simulink model "oldCubesatFullSim"  (R2024a)
settings: Solver=FixedStepAuto  StartTime=0.0  StopTime=7200  FixedStep=0.01  MaxStep=1  MinStep=0.001  RelTol=1e-3
libraries: sharedtransform x2, simulink_extras x2, aerolibutil x1
settings Model: Creator=samuel  LastModifiedBy=joshu
settings OptimizationCC: ReuseModelBlockBuffer=off
settings ModelReferenceCC: EnableRefExpFcnMdlSchedulingChecks=on
settings RTWCC: GPUComputeCapability=3.5

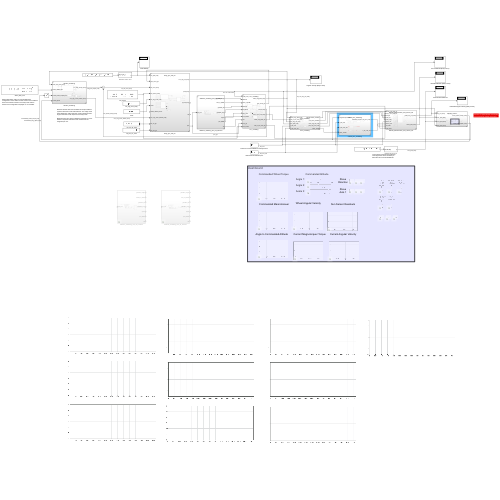
[thumbnail: Simulink's stored preview of the top-level diagram]
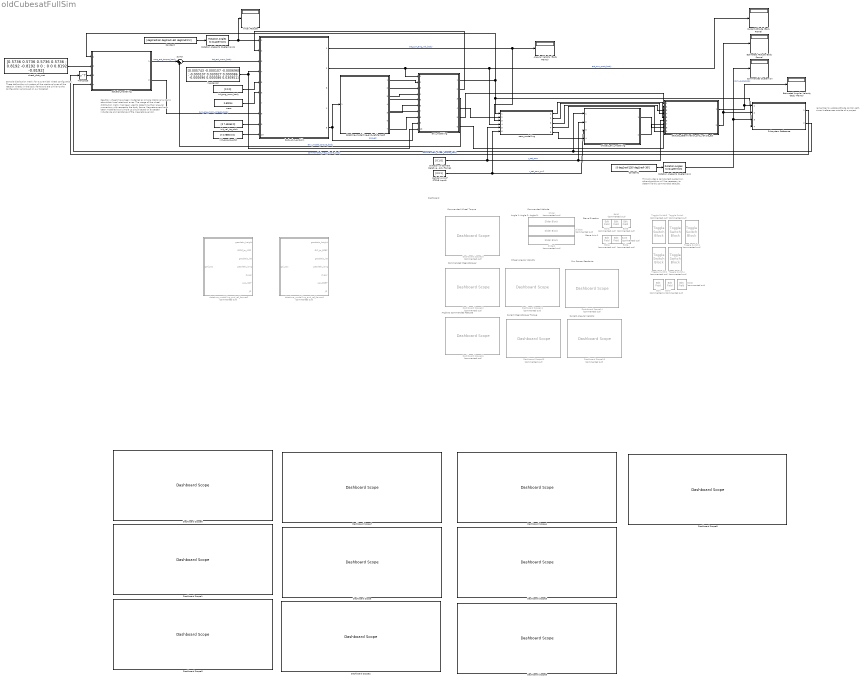
== system oldCubesatFullSim ==
  note: remember to update attitude control path,
      | since it references outside of a project
  note: This provides a sample test quaternion, other algorithms will be necessary to determine this commanded attitude.
  note: Reaction wheels have been modelled as simple rotational systems about their local rotational axes. The usage of the wheel distribution matrix has been used to determine their angular momentum with respect to the body frame.
      |
      | Magnetorquers have been modelled as a simple LC circuit based on expected inductance and resistance of the magnetorquer coil.
  note: Sample distribution matrix for a pyramidal wheel configuration. These define the unit vectors of the rotational axes of the reaction wheels in the body frame and are similar to the configuration employed on our CubeSat.
  note: Commanded Wheel Torque
  note: Angle to Commanded Attitude
  note: Dashboard
  note: Wheel Angular Velocity
  note: Commanded Attitude
  note: Commanded Magnotorquer
  note: Steve Axis 1
  note: Angle 1:
      |
      | Angle 2:
      |
      | Angle 3:
  note: Current Angular Velocity
  note: Steve Direction
  note: Current Magnotorquer Torque
  note: Sun Sensor Readouts
  Angular Velocity (Body Frame) : Display
  Commanded Quaternion : Display
  Constant : Constant  Value=[deg2rad(34) deg2rad(-63) deg2rad(21)]
  Constant1 : Constant  Value=[0 deg2rad(135) deg2rad(-30)]
  Current Attitude (Body Frame) : Display
  Dashboard Scope{,1..9} (10 alike) : DashboardScope
  Dashboard Scope10 : DashboardScope  Commented=on  Ymin=0  NormalizeYAxis=on  TicksPosition=Inside
  Dashboard Scope{11..15} (5 alike) : DashboardScope  Commented=on  TicksPosition=Inside
  Dashboard Scope16 : DashboardScope  Commented=on  Ymin=0  UpdateMode=Scroll  NormalizeYAxis=on  TicksPosition=Inside
  Direction of Camera Relative to Body Frame1 : Constant  Value=[0 1 0]
  Edit{,1..8} (9 alike) : EditField  Commented=on  LabelPosition=Hide  ShowInitialText=on  Alignment=Center
  Estimated Angular Velocity (Body Frame) : Display
  Estimated Attitude (Body Frame) : Display
  Initial Attitude : Display
  Rotation Angles to Quaternions : sharedtransform/Rotation Angles to Quaternions  rotationOrder=ZYX  aMode=aMode
  Rotation Angles to Quaternions1 : sharedtransform/Rotation Angles to Quaternions  rotationOrder=ZYX  aMode=aMode
  Slider : SliderBlock  Commented=on  LabelPosition=Hide  ScaleMin=-3.1415  ScaleMax=3.1415
  Slider1 : SliderBlock  Commented=on  LabelPosition=Hide  ScaleMin=-3.1415  ScaleMax=3.1415
  Slider2 : SliderBlock  Commented=on  LabelPosition=Hide  ScaleMin=-3.1415  ScaleMax=3.1415
  Subsystem Reference : Subsystem  ReferencedSubsystem=attitude_control
  Sum3 : Sum  Inputs=|++
  Toggle Switch{,1..4} (5 alike) : ToggleSwitchBlock  Commented=on
      settings: Values={{'Off', 'On'}, [0 1]}
  Transpose : Math  Operator=transpose
  Vertical Axis of STEVE Input1 : Constant  Value=[0 0 1]
  actuator_modelling : Subsystem  ReferencedSubsystem=actuator_modelling
  attitude_determination_and_vehicle_est : Subsystem  ReferencedSubsystem=attitude_determination_and_vehicle_est
  body_dyn_and_kin : Subsystem  ReferencedSubsystem=body_dyn_and_kin
  datetime_modelling_and_ref_frames1 : Subsystem  Commented=on
  datetime_modelling_and_ref_frames2 : Subsystem  Commented=on
  datetime_modelling_and_ref_frames3 : Subsystem  ReferencedSubsystem=datetime_modelling_and_ref_frames
  env_modelling : Subsystem  ReferencedSubsystem=env_modelling
  iner_tensor : Constant  Value=[0.005743 -0.000107 -0.0006965 ; -0.000107 0.030927 0.000086 ; -0.000696 0.000086 0.030951]
  init_ang_mom_body : Constant  Value=[0 0 0]
  init_pos_iss_orbit : Constant  Value=[7.178e6 0 0]
  init_vel_iss_orbit : Constant  Value=[0 7.452e3 0]
  mass : Constant  Value=2.60014
  onboad_env_modelling : Subsystem  ReferencedSubsystem=onboad_env_modelling
  sens_modelling : Subsystem  ReferencedSubsystem=sens_modelling
  wheel_distr_mat : Constant  Value=[0.5736 0.5736 0.5736 0.5736 ; 0.8192 -0.8192 0 0 ; 0 0 0.8192 -0.8192]
  wires:
  iner_tensor/1 -> env_modelling/10, body_dyn_and_kin/4
  wheel_distr_mat/1 -> actuator_modelling/2
  actuator_modelling/1 -> Sum3/1  "mag_act_torque_body"
  body_dyn_and_kin/2 -> sens_modelling/4, Current Attitude (Body Frame)/1, env_modelling/1  "act_curr_quat_body"
  body_dyn_and_kin/5 -> datetime_modelling_and_ref_frames3/1, env_modelling/9  "pos_gci"
  Sum3/1 -> body_dyn_and_kin/3  "tot_ext_mom_body"
  init_ang_mom_body/1 -> body_dyn_and_kin/5
  mass/1 -> body_dyn_and_kin/6
  actuator_modelling/2 -> body_dyn_and_kin/8  "curr_ang_mom_wheels_body"
  init_vel_iss_orbit/1 -> body_dyn_and_kin/9
  init_pos_iss_orbit/1 -> body_dyn_and_kin/10
  env_modelling/1 -> sens_modelling/1, Subsystem Reference/4, actuator_modelling/1
  datetime_modelling_and_ref_frames3/1 -> env_modelling/2
  datetime_modelling_and_ref_frames3/2 -> env_modelling/3
  datetime_modelling_and_ref_frames3/3 -> env_modelling/4
  datetime_modelling_and_ref_frames3/4 -> env_modelling/5
  datetime_modelling_and_ref_frames3/5 -> env_modelling/6
  datetime_modelling_and_ref_frames3/6 -> env_modelling/7
  datetime_modelling_and_ref_frames3/7 -> env_modelling/8
  env_modelling/2 -> body_dyn_and_kin/2
  env_modelling/3 -> Sum3/2  "env_model_torque_body"
  env_modelling/4 -> sens_modelling/2
  attitude_determination_and_vehicle_est/1 -> Estimated Angular Velocity (Body Frame)/1, Subsystem Reference/1
  attitude_determination_and_vehicle_est/2 -> Estimated Attitude (Body Frame)/1, Subsystem Reference/2
  Subsystem Reference/1 -> Transpose/1  "commanded_wheel_torque_body"
  body_dyn_and_kin/1 -> sens_modelling/3, Angular Velocity (Body Frame)/1  "act_curr_ang_vel_body"
  sens_modelling/1 -> attitude_determination_and_vehicle_est/5
  sens_modelling/2 -> attitude_determination_and_vehicle_est/4
  env_modelling/5 -> attitude_determination_and_vehicle_est/1
  env_modelling/6 -> attitude_determination_and_vehicle_est/2
  Transpose/1 -> actuator_modelling/3
  Constant1/1 -> Rotation Angles to Quaternions/1
  Rotation Angles to Quaternions/1 -> Subsystem Reference/3, Commanded Quaternion/1  "com_quat_body"
  Rotation Angles to Quaternions1/1 -> body_dyn_and_kin/1, Initial Attitude/1
  Constant/1 -> Rotation Angles to Quaternions1/1
  Subsystem Reference/2 -> actuator_modelling/4, onboad_env_modelling/1  "commanded_mag_dipole_body"
  Direction of Camera Relative to Body Frame1/1 -> onboad_env_modelling/2, attitude_determination_and_vehicle_est/6, sens_modelling/5  "r_sat_com"
  Vertical Axis of STEVE Input1/1 -> sens_modelling/6, onboad_env_modelling/3  "r_sat_com_ax1"
  sens_modelling/3 -> attitude_determination_and_vehicle_est/3
  sens_modelling/5 -> onboad_env_modelling/4
  onboad_env_modelling/2 -> attitude_determination_and_vehicle_est/7
  onboad_env_modelling/1 -> attitude_determination_and_vehicle_est/8
  sens_modelling/4 -> attitude_determination_and_vehicle_est/9

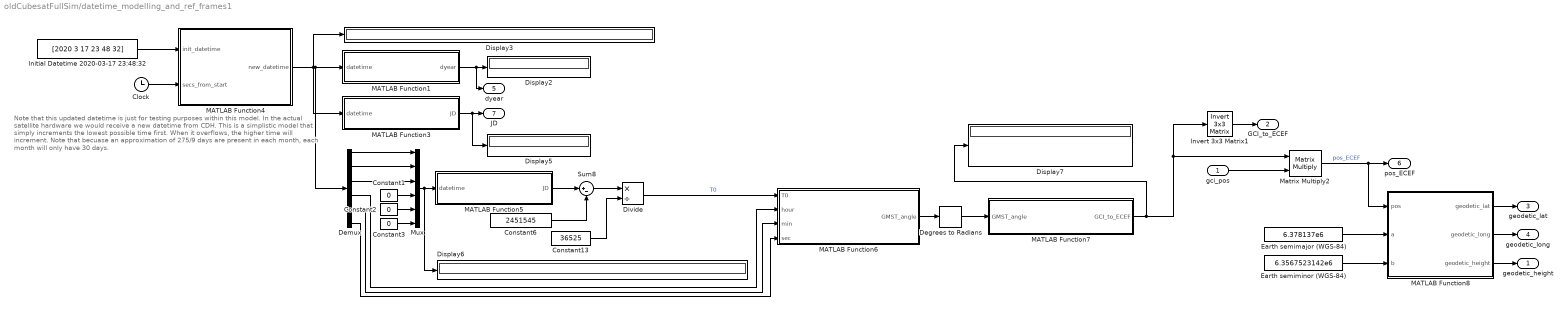
== system oldCubesatFullSim/datetime_modelling_and_ref_frames1 ==
  note: Note that this updated datetime is just for testing purposes within this model. In the actual satellite hardware we would receive a new datetime from CDH. This is a simplistic model that simply increments the lowest possible time first. When it overflows, the higher time will increment. Note that becuase an approximation of 275/9 days are present in each month, each month will only have 30 days.
  gci_pos : Inport
  Clock : Clock
  Constant1 : Constant  Value=0
  Constant13 : Constant  Value=36525
  Constant2 : Constant  Value=0
  Constant3 : Constant  Value=0
  Constant6 : Constant  Value=2451545
  Degrees to Radians : simulink_extras/Transformations/Degrees to Radians
  Demux : Demux  Outputs=6
  Display{2..3,5..7} (5 alike) : Display
  Divide : Product  Inputs=*/
  Earth semimajor (WGS-84) : Constant  Value=6.378137e6
  Earth semiminor (WGS-84) : Constant  Value=6.3567523142e6
  Initial Datetime 2020-03-17 23:48:32 : Constant  Value=[2020 3 17 23 48 32]
  Invert 3x3 Matrix1 : aerolibutil/Invert  3x3 Matrix
  MATLAB Function1 : MATLAB Function  TreatAsAtomicUnit=on
  MATLAB Function3 : MATLAB Function  TreatAsAtomicUnit=on
  MATLAB Function4 : MATLAB Function  TreatAsAtomicUnit=on
  MATLAB Function5 : MATLAB Function  TreatAsAtomicUnit=on
  MATLAB Function6 : MATLAB Function  TreatAsAtomicUnit=on
  MATLAB Function7 : MATLAB Function  TreatAsAtomicUnit=on
  MATLAB Function8 : MATLAB Function  TreatAsAtomicUnit=on
  Matrix Multiply2 : Product  Multiplication=Matrix(*)
  Mux : Mux  Inputs=6
  Sum8 : Sum  Inputs=|+-
  geodetic_height : Outport
  GCI_to_ECEF : Outport  Port=2
  geodetic_lat : Outport  Port=3
  geodetic_long : Outport  Port=4
  dyear : Outport  Port=5
  pos_ECEF : Outport  Port=6
  JD : Outport  Port=7
  wires:
  Constant3/1 -> Mux/6
  MATLAB Function8/1(geodetic_lat) -> geodetic_lat/1
  Divide/1 -> MATLAB Function6/1(T0)  "T0"
  MATLAB Function4/1(new_datetime) -> Demux/1, MATLAB Function1/1(datetime), MATLAB Function3/1(datetime), Display3/1
  MATLAB Function6/1(GMST_angle) -> Degrees to Radians/1
  MATLAB Function1/1(dyear) -> dyear/1, Display2/1
  Invert 3x3 Matrix1/1 -> GCI_to_ECEF/1
  MATLAB Function3/1(JD) -> Display5/1, JD/1
  MATLAB Function8/3(geodetic_height) -> geodetic_height/1
  MATLAB Function8/2(geodetic_long) -> geodetic_long/1
  Constant1/1 -> Mux/4
  Demux/5 -> MATLAB Function6/3(min)
  Demux/1 -> Mux/1
  Sum8/1 -> Divide/1
  Constant13/1 -> Divide/2
  Earth semiminor (WGS-84)/1 -> MATLAB Function8/3(b)
  Earth semimajor (WGS-84)/1 -> MATLAB Function8/2(a)
  Matrix Multiply2/1 -> MATLAB Function8/1(pos), pos_ECEF/1  "pos_ECEF"
  Demux/6 -> MATLAB Function6/4(sec)
  Constant6/1 -> Sum8/2
  gci_pos/1 -> Matrix Multiply2/2
  MATLAB Function5/1(JD) -> Sum8/1
  MATLAB Function7/1(GCI_to_ECEF) -> Matrix Multiply2/1, Invert 3x3 Matrix1/1, Display7/1
  Degrees to Radians/1 -> MATLAB Function7/1(GMST_angle)
  Mux/1 -> Display6/1, MATLAB Function5/1(datetime)
  Initial Datetime 2020-03-17 23:48:32/1 -> MATLAB Function4/1(init_datetime)
  Clock/1 -> MATLAB Function4/2(secs_from_start)
  Demux/3 -> Mux/3
  Demux/4 -> MATLAB Function6/2(hour)
  Demux/2 -> Mux/2
  Constant2/1 -> Mux/5

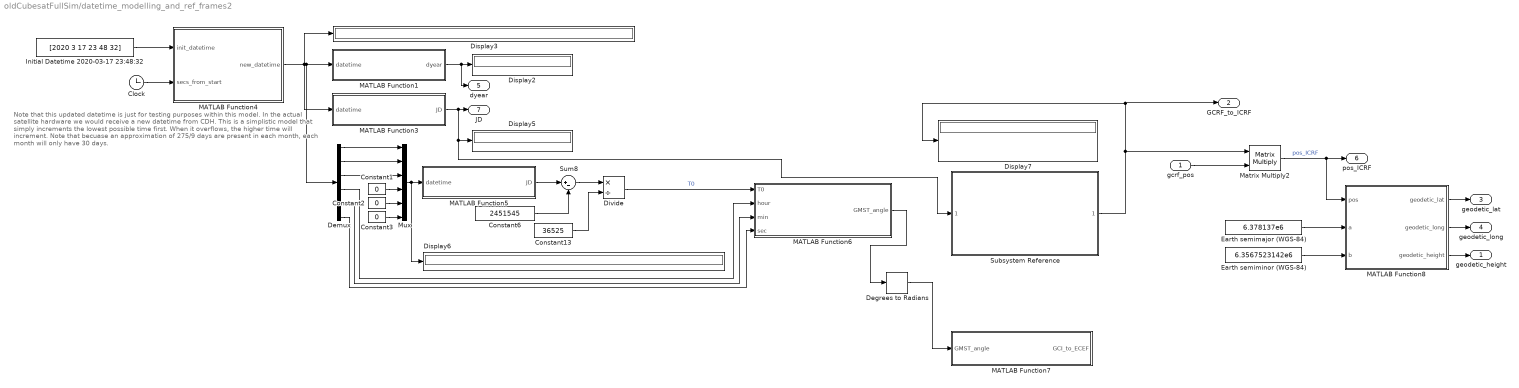
== system oldCubesatFullSim/datetime_modelling_and_ref_frames2 ==
  note: Note that this updated datetime is just for testing purposes within this model. In the actual satellite hardware we would receive a new datetime from CDH. This is a simplistic model that simply increments the lowest possible time first. When it overflows, the higher time will increment. Note that becuase an approximation of 275/9 days are present in each month, each month will only have 30 days.
  gcrf_pos : Inport
  Clock : Clock
  Constant1 : Constant  Value=0
  Constant13 : Constant  Value=36525
  Constant2 : Constant  Value=0
  Constant3 : Constant  Value=0
  Constant6 : Constant  Value=2451545
  Degrees to Radians : simulink_extras/Transformations/Degrees to Radians
  Demux : Demux  Outputs=6
  Display{2..3,5..7} (5 alike) : Display
  Divide : Product  Inputs=*/
  Earth semimajor (WGS-84) : Constant  Value=6.378137e6
  Earth semiminor (WGS-84) : Constant  Value=6.3567523142e6
  Initial Datetime 2020-03-17 23:48:32 : Constant  Value=[2020 3 17 23 48 32]
  MATLAB Function1 : MATLAB Function  TreatAsAtomicUnit=on
  MATLAB Function3 : MATLAB Function  TreatAsAtomicUnit=on
  MATLAB Function4 : MATLAB Function  TreatAsAtomicUnit=on
  MATLAB Function5 : MATLAB Function  TreatAsAtomicUnit=on
  MATLAB Function6 : MATLAB Function  TreatAsAtomicUnit=on
  MATLAB Function7 : MATLAB Function  TreatAsAtomicUnit=on
  MATLAB Function8 : MATLAB Function  TreatAsAtomicUnit=on
  Matrix Multiply2 : Product  Multiplication=Matrix(*)
  Mux : Mux  Inputs=6
  Subsystem Reference : Subsystem  ReferencedSubsystem=GCRF_to_ICRF
  Sum8 : Sum  Inputs=|+-
  geodetic_height : Outport
  GCRF_to_ICRF : Outport  Port=2
  geodetic_lat : Outport  Port=3
  geodetic_long : Outport  Port=4
  dyear : Outport  Port=5
  pos_ICRF : Outport  Port=6
  JD : Outport  Port=7
  wires:
  Constant3/1 -> Mux/6
  MATLAB Function8/1(geodetic_lat) -> geodetic_lat/1
  Divide/1 -> MATLAB Function6/1(T0)  "T0"
  MATLAB Function4/1(new_datetime) -> Demux/1, MATLAB Function1/1(datetime), MATLAB Function3/1(datetime), Display3/1
  MATLAB Function6/1(GMST_angle) -> Degrees to Radians/1
  MATLAB Function1/1(dyear) -> dyear/1, Display2/1
  MATLAB Function3/1(JD) -> Subsystem Reference/1, Display5/1, JD/1
  MATLAB Function8/3(geodetic_height) -> geodetic_height/1
  MATLAB Function8/2(geodetic_long) -> geodetic_long/1
  Constant1/1 -> Mux/4
  Demux/5 -> MATLAB Function6/3(min)
  Demux/1 -> Mux/1
  Sum8/1 -> Divide/1
  Constant13/1 -> Divide/2
  Earth semiminor (WGS-84)/1 -> MATLAB Function8/3(b)
  Earth semimajor (WGS-84)/1 -> MATLAB Function8/2(a)
  Matrix Multiply2/1 -> MATLAB Function8/1(pos), pos_ICRF/1  "pos_ICRF"
  Demux/6 -> MATLAB Function6/4(sec)
  Constant6/1 -> Sum8/2
  gcrf_pos/1 -> Matrix Multiply2/2
  MATLAB Function5/1(JD) -> Sum8/1
  Degrees to Radians/1 -> MATLAB Function7/1(GMST_angle)
  Mux/1 -> Display6/1, MATLAB Function5/1(datetime)
  Initial Datetime 2020-03-17 23:48:32/1 -> MATLAB Function4/1(init_datetime)
  Clock/1 -> MATLAB Function4/2(secs_from_start)
  Demux/3 -> Mux/3
  Demux/4 -> MATLAB Function6/2(hour)
  Demux/2 -> Mux/2
  Constant2/1 -> Mux/5
  Subsystem Reference/1 -> Matrix Multiply2/1, GCRF_to_ICRF/1, Display7/1

== matlab function oldCubesatFullSim/datetime_modelling_and_ref_frames2/MATLAB Function7 ==
  data: GMST_angle input; GCI_to_ECEF output
function GCI_to_ECEF = calc_GCI_to_ECEF_from_GMST_angle(GMST_angle)

% calculates the transformation matrix from GCI to ECEF
GCI_to_ECEF = [cos(GMST_angle) sin(GMST_angle) 0 ; ...
    -sin(GMST_angle) cos(GMST_angle) 0 ; 0 0 1];

== matlab function oldCubesatFullSim/datetime_modelling_and_ref_frames2/MATLAB Function8 ==
  data: pos input; geodetic_lat output; a input; b input; geodetic_long output; geodetic_height output
function [geodetic_lat, geodetic_long, geodetic_height] = ...
    ECEF_coords_to_geodetic(pos, a, b)

    % converts from ECEF coordinates to geodetic coordinates

    x = pos(1);
    y = pos(2);
    z = pos(3);

    e2 = 1 - b^2 / a^2;
    eps2 = a^2 / b^2 - 1;
    rho = sqrt(x^2 + y^2);

    p = abs(z)/eps2;
    s = rho^2/(e2*eps2);
    q = p^2 - b^2 + s;

    u = p/sqrt(q);
    v = b^2*u^2/q;
    P=27*v*s/q;
    Q=(sqrt(P+1) + sqrt(P))^(2/3);

    t=(1+Q+1/Q)/6;
    c=sqrt(u^2-1+2*t);
    w=(c-u)/2;

    d=sign(z)*sqrt(q)*(w+sqrt(t^2+v)-u*w-t/2-1/4);

    N = a*sqrt(1+eps2*d^2/b^2);
    lat = asin((eps2+1)*(d/N));
    
    h = rho*cos(lat)+z*sin(lat)-a^2/N;
    long = atan2(y, x);

    % converts from rad to deg
    geodetic_lat = rad2deg(lat);
    geodetic_long = rad2deg(long);

    geodetic_height = h;

== matlab function oldCubesatFullSim/datetime_modelling_and_ref_frames1/MATLAB Function1 ==
  data: datetime input; dyear output
function dyear = dyear_from_datetime(datetime)

    % the datetime format is provided as a 6 value array
    % year, month, day, hour, minute, second

    % sequentially builds the decimal year

    % potentially we may want to use /61 for leap second days but this is
    % likely fine as our simulation just needs to perform regular datetime
    % updates for simple testing

    tot_mins = datetime(5) + datetime(6) / 60;
    tot_hours = datetime(4) + tot_mins / 60;
    tot_days = datetime(3) + tot_hours / 24;
    tot_months = datetime(2) + tot_days / (275/9); % average days in month across year
    tot_years = datetime(1) + tot_months / 12;

    dyear = tot_years;

== matlab function oldCubesatFullSim/datetime_modelling_and_ref_frames1/MATLAB Function3 ==
  data: datetime input; JD output
function JD = calc_JD_from_datetime(datetime)

% the datetime format is provided as a 6 value array
% year, month, day, hour, minute, second

% calculates the Julian date (JD) from the datetime
JD = 1721013.5 + 367*datetime(1) - floor(7/4*(datetime(1) + ...
    floor((datetime(2) + 9)/12))) + floor(275/9*datetime(2)) + ...
    datetime(3) + (60*datetime(4) + datetime(5) + datetime(6)/60)/1440;

% note that seconds should be /61 for leap days but since we are using a
% testing environment we do not need to worry about this

% presumably in the navigation system of the actual satellite we may also
% not need to consider this as it would introduce a negligible error or we
% may need to have some special protocol with CDH to figure out a system

== matlab function oldCubesatFullSim/datetime_modelling_and_ref_frames1/MATLAB Function4 ==
  data: init_datetime input; new_datetime output; secs_from_start input
function new_datetime  = datetime_upd(init_datetime, secs_from_start)

% the datetime format is provided as a 6 value array
% year, month, day, hour, minute, second

% initializes new datetime array
new_datetime = zeros(1, 6);

% adds the seconds from start of simulation to seconds
new_datetime(6) = init_datetime(6) + secs_from_start;

% computes the new seconds and minutes with carry over
new_datetime(5) = init_datetime(5) + floor(new_datetime(6) / 60);
new_datetime(6) = mod(new_datetime(6), 60);

% computes the new minutes and hours with carry over
new_datetime(4) = init_datetime(4) + floor(new_datetime(5) / 60);
new_datetime(5) = mod(new_datetime(5), 60);

% computes the new hours and days with carry over
new_datetime(3) = init_datetime(3) + floor(new_datetime(4) / 24);
new_datetime(4) = mod(new_datetime(4), 24);

% computes the new days and months with carry over
new_datetime(2) = init_datetime(2) + floor(new_datetime(3) / (275/9));

% NOTE: the floor here is specifically needed to prevent a recurring
% decimal from occurring here due to using an average number of days per
% month of 275/9 (this also caps days in a month to 30)
new_datetime(3) = floor(mod(new_datetime(3), (275/9)));

% computes the new months and years with carry over

% for calculations, shifts first month to 0
new_datetime(2) = new_datetime(2) - 1;

new_datetime(1) = init_datetime(1) + floor(new_datetime(2) / 12);

% done with calculations, restores first month to 1
new_datetime(2) = mod(new_datetime(2), 12) + 1;

end

== matlab function oldCubesatFullSim/datetime_modelling_and_ref_frames1/MATLAB Function5 ==
  data: datetime input; JD output
function JD = calc_JD_from_datetime(datetime)

% the datetime format is provided as a 6 value array
% year, month, day, hour, minute, second

% calculates the Julian date (JD) from the datetime
JD = 1721013.5 + 367*datetime(1) - floor(7/4*(datetime(1) + ...
    floor((datetime(2) + 9)/12))) + floor(275/9*datetime(2)) + ...
    datetime(3) + (60*datetime(4) + datetime(5) + datetime(6)/60)/1440;

% note that seconds should be /61 for leap days but since we are using a
% testing environment we do not need to worry about this

% presumably in the navigation system of the actual satellite we may also
% not need to consider this as it would introduce a negligible error or we
% may need to have some special protocol with CDH to figure out a system

== matlab function oldCubesatFullSim/datetime_modelling_and_ref_frames1/MATLAB Function6 ==
  data: T0 input; GMST_angle output; hour input; min input; sec input
function GMST_angle = calc_GMST_angle_from_T0(T0, hour, min, sec)

% calculates GMST_angle in units of seconds (longitudinal seconds)
GMST_angle = 24110.54841 + 8640184.812866 * T0 + 0.093104 * T0^2 ...
    - 6.2e-6 * T0^3 + 1.002737909350795 * (3600*hour + 60*min + sec);

% reduces to range of 0-86400
GMST_angle = mod(GMST_angle, 86400);

% converts to degrees (there are 240 longitudinal seconds in a degree)
GMST_angle = GMST_angle / 240;

== matlab function oldCubesatFullSim/datetime_modelling_and_ref_frames1/MATLAB Function7 ==
  data: GMST_angle input; GCI_to_ECEF output
function GCI_to_ECEF = calc_GCI_to_ECEF_from_GMST_angle(GMST_angle)

% calculates the transformation matrix from GCI to ECEF
GCI_to_ECEF = [cos(GMST_angle) sin(GMST_angle) 0 ; ...
    -sin(GMST_angle) cos(GMST_angle) 0 ; 0 0 1];

== matlab function oldCubesatFullSim/datetime_modelling_and_ref_frames1/MATLAB Function8 ==
  data: pos input; geodetic_lat output; a input; b input; geodetic_long output; geodetic_height output
function [geodetic_lat, geodetic_long, geodetic_height] = ...
    ECEF_coords_to_geodetic(pos, a, b)

    % converts from ECEF coordinates to geodetic coordinates

    x = pos(1);
    y = pos(2);
    z = pos(3);

    e2 = 1 - b^2 / a^2;
    eps2 = a^2 / b^2 - 1;
    rho = sqrt(x^2 + y^2);

    p = abs(z)/eps2;
    s = rho^2/(e2*eps2);
    q = p^2 - b^2 + s;

    u = p/sqrt(q);
    v = b^2*u^2/q;
    P=27*v*s/q;
    Q=(sqrt(P+1) + sqrt(P))^(2/3);

    t=(1+Q+1/Q)/6;
    c=sqrt(u^2-1+2*t);
    w=(c-u)/2;

    d=sign(z)*sqrt(q)*(w+sqrt(t^2+v)-u*w-t/2-1/4);

    N = a*sqrt(1+eps2*d^2/b^2);
    lat = asin((eps2+1)*(d/N));
    
    h = rho*cos(lat)+z*sin(lat)-a^2/N;
    long = atan2(y, x);

    % converts from rad to deg
    geodetic_lat = rad2deg(lat);
    geodetic_long = rad2deg(long);

    geodetic_height = h;

== matlab function oldCubesatFullSim/datetime_modelling_and_ref_frames2/MATLAB Function1 ==
  data: datetime input; dyear output
function dyear = dyear_from_datetime(datetime)

    % the datetime format is provided as a 6 value array
    % year, month, day, hour, minute, second

    % sequentially builds the decimal year

    % potentially we may want to use /61 for leap second days but this is
    % likely fine as our simulation just needs to perform regular datetime
    % updates for simple testing

    tot_mins = datetime(5) + datetime(6) / 60;
    tot_hours = datetime(4) + tot_mins / 60;
    tot_days = datetime(3) + tot_hours / 24;
    tot_months = datetime(2) + tot_days / (275/9); % average days in month across year
    tot_years = datetime(1) + tot_months / 12;

    dyear = tot_years;

== matlab function oldCubesatFullSim/datetime_modelling_and_ref_frames2/MATLAB Function3 ==
  data: datetime input; JD output
function JD = calc_JD_from_datetime(datetime)

% the datetime format is provided as a 6 value array
% year, month, day, hour, minute, second

% calculates the Julian date (JD) from the datetime
JD = 1721013.5 + 367*datetime(1) - floor(7/4*(datetime(1) + ...
    floor((datetime(2) + 9)/12))) + floor(275/9*datetime(2)) + ...
    datetime(3) + (60*datetime(4) + datetime(5) + datetime(6)/60)/1440;

% note that seconds should be /61 for leap days but since we are using a
% testing environment we do not need to worry about this

% presumably in the navigation system of the actual satellite we may also
% not need to consider this as it would introduce a negligible error or we
% may need to have some special protocol with CDH to figure out a system

== matlab function oldCubesatFullSim/datetime_modelling_and_ref_frames2/MATLAB Function4 ==
  data: init_datetime input; new_datetime output; secs_from_start input
function new_datetime  = datetime_upd(init_datetime, secs_from_start)

% the datetime format is provided as a 6 value array
% year, month, day, hour, minute, second

% initializes new datetime array
new_datetime = zeros(1, 6);

% adds the seconds from start of simulation to seconds
new_datetime(6) = init_datetime(6) + secs_from_start;

% computes the new seconds and minutes with carry over
new_datetime(5) = init_datetime(5) + floor(new_datetime(6) / 60);
new_datetime(6) = mod(new_datetime(6), 60);

% computes the new minutes and hours with carry over
new_datetime(4) = init_datetime(4) + floor(new_datetime(5) / 60);
new_datetime(5) = mod(new_datetime(5), 60);

% computes the new hours and days with carry over
new_datetime(3) = init_datetime(3) + floor(new_datetime(4) / 24);
new_datetime(4) = mod(new_datetime(4), 24);

% computes the new days and months with carry over
new_datetime(2) = init_datetime(2) + floor(new_datetime(3) / (275/9));

% NOTE: the floor here is specifically needed to prevent a recurring
% decimal from occurring here due to using an average number of days per
% month of 275/9 (this also caps days in a month to 30)
new_datetime(3) = floor(mod(new_datetime(3), (275/9)));

% computes the new months and years with carry over

% for calculations, shifts first month to 0
new_datetime(2) = new_datetime(2) - 1;

new_datetime(1) = init_datetime(1) + floor(new_datetime(2) / 12);

% done with calculations, restores first month to 1
new_datetime(2) = mod(new_datetime(2), 12) + 1;

end

== matlab function oldCubesatFullSim/datetime_modelling_and_ref_frames2/MATLAB Function5 ==
  data: datetime input; JD output
function JD = calc_JD_from_datetime(datetime)

% the datetime format is provided as a 6 value array
% year, month, day, hour, minute, second

% calculates the Julian date (JD) from the datetime
JD = 1721013.5 + 367*datetime(1) - floor(7/4*(datetime(1) + ...
    floor((datetime(2) + 9)/12))) + floor(275/9*datetime(2)) + ...
    datetime(3) + (60*datetime(4) + datetime(5) + datetime(6)/60)/1440;

% note that seconds should be /61 for leap days but since we are using a
% testing environment we do not need to worry about this

% presumably in the navigation system of the actual satellite we may also
% not need to consider this as it would introduce a negligible error or we
% may need to have some special protocol with CDH to figure out a system

== matlab function oldCubesatFullSim/datetime_modelling_and_ref_frames2/MATLAB Function6 ==
  data: T0 input; GMST_angle output; hour input; min input; sec input
function GMST_angle = calc_GMST_angle_from_T0(T0, hour, min, sec)

% calculates GMST_angle in units of seconds (longitudinal seconds)
GMST_angle = 24110.54841 + 8640184.812866 * T0 + 0.093104 * T0^2 ...
    - 6.2e-6 * T0^3 + 1.002737909350795 * (3600*hour + 60*min + sec);

% reduces to range of 0-86400
GMST_angle = mod(GMST_angle, 86400);

% converts to degrees (there are 240 longitudinal seconds in a degree)
GMST_angle = GMST_angle / 240;
